simulink model "Car_boundary_testingDec_27_downsample_2012b"  (Simulink 8.0)
settings: Solver=ode5  StartTime=0.0  StopTime=inf  FixedStep=sample_time  RelTol=1e-3
InitFcn:
  | sample_time=0.005;%0.004;%0.0025;%0.02;
  | sample_time_Vicon = 0.005;
  | DeltaT = 0.02;
  | g = 9.81;
  | H0 = g%0.3165;
  | Kl = 1;
  | 
  | Q6_mass = 0.825;
  | 
  | Q6_Omega_r = 1.5; %for horizon ref
  | Q6_Zeta_r = 0.5; %for horizon ref
  | Q6_Omega_r_h = 2;%for vertical ref
  | Q6_Zeta_r_h = 1; %for vertical ref
  | 
  | 
  | Q6_Omega = 1.5; %for horizon control
  | Q6_Zeta = 0.5; %for horizon control
  | Q6_Omega_h= 2; %for vertical control
  | Q6_Zeta_h = 0.7; %for vertical control
  | 
  | 
  | Q6_acc_max = 5;%horizontal max acc
  | Q6_acc_max_h = 3;%horizontal max acc
  | 
  | omega_circle = 72*pi/180;
  | omega_h = 0.1;%Ascending speed
  | PI = pi;
  | Circle_R = 2.5;
  | MAX_Height = -2;
undefined symbols (not defined in the file): DiscIntNeverNeededParam
libraries: simulink x13, X330_Control x5, commsequence2 x5
(part 2 of 2)

== stateflow chart UAV 1/Trajectory Logic/UAV SF1 ==
  state Landing
    state Decsending
      en:PosDesired = Pos;
      du:PosDesired[2] = (0 - PosDesired[2])*1*DeltaT + PosDesired[2] ;
    state CutThrottle
      du:HoverThrottle = (0.01 - HoverThrottle)*2*DeltaT + HoverThrottle ;
    (default) -> Decsending
    Decsending -> CutThrottle : [Pos[2] > -0.15]
  state Airborne1
    state TakeOff
      du:HoverThrottle = (H0 - HoverThrottle)*2*DeltaT + HoverThrottle ;
    state Hover
      en: PosDesired[2] = -1;
    state capturing_sequence
      state normal_capturing
        en: PosDesired[0] = carest[0]; PosDesired[1] = carest[1]; PosDesired[2] = -0.8
        ex: after(5,sec);
        normal_capturing -> normal_capturing [order 1] : [match_flag==0]
      state success_capturing
        en: PosDesired[0] = Pos[0];PosDesired[1] = Pos[1]; PosDesired[2] = -1.7;
        ex: after(5,sec);
      state capture_landing
        state Decsending1
          en:PosDesired[0] = Pos[0]; PosDesired[1] = Pos[1]; PosDesired[2] = Pos[2]; PosDesired[3] = landing_area[3]
          du:PosDesired[2] = (0 - PosDesired[2])*1*DeltaT + PosDesired[2] ;
        state CutThrottle1
          du:HoverThrottle = (0.01 - HoverThrottle)*2*DeltaT + HoverThrottle ;
        (default) -> Decsending1
        Decsending1 -> CutThrottle1 : [Pos[2] > (landing_area[3]  - 0.2)]
      state Move_to_landing_area
        du: PosDesired[0] = Pos[0]; PosDesired[1] = Pos[1]; PosDesired[2] = -0.8 + landing_area[2];
      state Move_to_landing_area1
        du: PosDesired[0] = landing_area[0]; PosDesired[1] = landing_area[1]; PosDesired[2] = -0.8 + landing_area[2]; PosDesired[3] = landing_area[5]
      success_capturing -> normal_capturing [order 1] : [(car[2] > -0.15)]
      (default) -> normal_capturing
      normal_capturing -> success_capturing [order 1] : [match_flag == 1]
      Move_to_landing_area -> normal_capturing [order 2] : [match_flag==0]
      success_capturing -> Move_to_landing_area [order 2] : [(stable_flag == 1)&(car[2]<-0.15)]
          | {smoothflag == 1;}
      Move_to_landing_area -> Move_to_landing_area [order 3] : [stable_flag == 0]
      Move_to_landing_area -> Move_to_landing_area1 [order 1] : after(10,sec)
      Move_to_landing_area1 -> capture_landing : [stable_flag == 1]
          | {HoverThrottle = 0.01;}
    (default) -> TakeOff : {PosDesired = Pos;  PosDesired[2] = -1;}
    Hover -> capturing_sequence : [RC[5] > 0]
    TakeOff -> Hover : after(5,sec)
        | {PosDesired = Pos;}
    capturing_sequence -> Hover : [RC[5] < 0]
        | {PosDesired = Pos;}
  Landing -> Airborne1 : [RC[6] > 0.5]
  Airborne1 -> Landing : [RC[6] < -0.5]
  (default) -> Landing : {HoverThrottle=0.01;}
  data: PosDesired output double size=4; HoverThrottle output double size=1; Mode output uint8 size=3; RC input double size=8; Pos input double size=4; DeltaT parameter double size=1; H0 parameter double size=1; Kl parameter double size=1; VelCmd local double size=2 =0; line_count local int8 size=1 =0; triangle_count local int8 size=1 =0; T_circle local double size=1; omega_circle parameter double size=1; PI parameter double size=1; omega_h parameter double; Circle_R parameter double size=1; MAX_Height parameter double size=1; carest input double size=2; car input double size=12; landing_area input double size=6; stable_flag input boolean size=1; match_flag input double; smoothflag output boolean size=1 [0..1] =0

== matlab function UAV 1/Trajectory Logic/stable_chk/stablize_checking ==
  data: posx input double; stable_flag output double; posy input double; carx input double; cary input double
function stable_flag = fcn(posx,posy,carx,cary)
%#codegen
subx = abs(posx - carx);
suby = abs(posy - cary);
if(subx < 0.1 && suby < 0.1)
    stable_flag = 1;
else
    stable_flag = 0;
end

== matlab function UAV 1/Trajectory Logic/Subsystem/match_chk ==
  data: vsx input double; match_flag output double; vsy input double
function match_flag = fcn(vsx,vsy)
%#codegen
if(abs(vsx) < 0.2 && abs(vsy) < 0.2)
    match_flag = 1;
else
    match_flag = 0;
end

== stateflow chart UAV 1/Trajectory Logic/UAV SF2 ==
  state Landing
    state Decsending
      en:PosDesired = Pos;
      du:PosDesired[2] = (0 - PosDesired[2])*1*DeltaT + PosDesired[2] ;
    state CutThrottle
      du:HoverThrottle = (0.01 - HoverThrottle)*2*DeltaT + HoverThrottle ;
    (default) -> Decsending
    Decsending -> CutThrottle : [Pos[2] > -0.15]
  state Airborne1
    state TakeOff
      du:HoverThrottle = (H0 - HoverThrottle)*2*DeltaT + HoverThrottle ;
    state capturing_sequence
      state normal_capturing1
        du: PosDesired[0] = carest[0]; PosDesired[1] = carest[1]; PosDesired[2] = -1.3;
      (default) -> normal_capturing1
    state Hover
      en: PosDesired[2] = -1;
    (default) -> TakeOff : {PosDesired = Pos;  PosDesired[2] = -1;}
    Hover -> capturing_sequence : [RC[5] > 0]
    TakeOff -> Hover : after(5,sec)
        | {PosDesired = Pos;}
    capturing_sequence -> Hover : [RC[5] < 0]
        | {PosDesired = Pos;}
  state normal_capturing
    en: PosDesired[0] = carest[0]; PosDesired[1] = carest[1]; PosDesired[2] = -1;
  state success_capturing
    en: PosDesired[0] = car[0];PosDesired[1] = car[1]; PosDesired[2] = -1.3;
  Landing -> Airborne1 : [RC[6] > 0.5]
  Airborne1 -> Landing : [RC[6] < -0.5]
  (default) -> Landing : {HoverThrottle=0.01;}
  data: PosDesired output double size=4; HoverThrottle output double size=1; Mode output uint8 size=3; RC input double size=8; Pos input double size=4; DeltaT parameter double size=1; H0 parameter double size=1; Kl parameter double size=1; VelCmd local double size=2 =0; line_count local int8 size=1 =0; triangle_count local int8 size=1 =0; T_line local double size=1; omega_circle parameter double size=1; PI parameter double size=1; omega_h parameter double; Circle_R parameter double size=1; MAX_Height parameter double size=1; carest input double size=2; car input double size=12; landing_area input double size=6; stable_flag input boolean size=1; match_flag input double; smoothflag output boolean size=1 [0..1] =0; transvec input double size=2; caroutbound input double size=1

== matlab function UAV 1/Trajectory Logic/Estimation_Subsystem/special_case_disablecirlin ==
  data: outbound input double; st_flag input double; estpx input double; estpy input double; estlinx input double; estliny input double; cirx output double; ciry output double; linx output double; liny output double; encir input double; enlin input double; ctrsig output double
function [cirx,ciry,linx,liny,ctrsig] = fcn(outbound, st_flag,estpx,estpy,estlinx,estliny,encir,enlin)
%#codegen
if(outbound == 1)
    cirx = 0;
    ciry = 0;
    linx = 0;
    liny = 0;
    ctrsig = 3;
else
    if(st_flag == 1)
        cirx = 0;
        ciry = 0;
        linx = 0;
        liny = 0;
        ctrsig = 4;
    else
        if(encir == 1)
        cirx = estpx;
        ciry = estpy;
        linx = 0;
        liny = 0;
        ctrsig = 1;
        else
            if(enlin == 1)
                 cirx = 0;
                 ciry = 0;
                 linx = estlinx;
                 liny = estliny;
                 ctrsig = 2;
            else
                cirx = 0;
                ciry = 0;
                linx = 0;
                liny = 0;
                ctrsig = 5;
            end
        end
      
    end
end

== matlab function UAV 1/Trajectory Logic/Estimation_Subsystem/boundary_chk1 ==
  data: boundedx output double; x input double; y input double; boundedy output double
function [boundedx,boundedy]  = fcn(x,y)
%#codegen

% define the boundry of a and b
%{
if (x < -3)  
    boundedx = -3;
elseif (x > 3)
    boundedx = 3;
elseif (x > landing_areax - 1.45 && y > landing_areay -1.45)
    boundedx = landing_areax - 1.45;
else
    boundedx = x;
end

if (y < -3)
    boundedy = -3;
elseif (y > 3)
      boundedy = 3;
elseif(x > landing_areax - 1.45 && y > landing_areay -1.45)
    boundedy = landing_areay - 1.45;
else
    boundedy = y;
    
end
%}
boundedx = x;
boundedy = y;

== matlab function UAV 1/Trajectory Logic/Estimation_Subsystem/MATLAB Function1 ==
  data: vx input double; magvel output double; vy input double
function magvel = fcn(vx,vy)
%#codegen
magvel = sqrt((vx)^2 + (vy)^2);

== matlab function UAV 1/Trajectory Logic/Estimation_Subsystem/MATLAB Function2 ==
  data: tranvecx input double; tranvecy input double; gain input double; x input double; y input double; Gx output double; Gy output double; st_flag input double; t input double; carx input double; cary input double
function [Gx,Gy] = fcn(tranvecx,tranvecy,gain,x,y,st_flag,t,carx,cary)
%#codegen
if(t<=2)
    Gx = carx;
    Gy = cary;
else
if(st_flag == 0)
magtran = sqrt(tranvecx^2 + tranvecy^2);
unit_tranvecx = tranvecx/magtran;
unit_tranvecy = tranvecy/magtran;
Gx = gain * unit_tranvecx + x;
Gy = gain * unit_tranvecy + y;
else
    Gx = carx;
    Gy = cary;
end
end

== matlab function UAV 1/Trajectory Logic/MATLAB Function2 ==
  data: tranvecx input double; tranvecy input double; x input double; y input double; Gx output double; Gy output double; st_flag input double; carx input double; cary input double
function [Gx,Gy] = fcn(tranvecx,tranvecy,x,y,st_flag,carx,cary)
%#codegen

if(st_flag == 0)
magtran = sqrt(tranvecx^2 + tranvecy^2);
unit_tranvecx = tranvecx/magtran;
unit_tranvecy = tranvecy/magtran;
Gx = 2 * unit_tranvecx + x;
Gy = 2 * unit_tranvecy + y;
else
    Gx = carx;
    Gy = cary;
end
